simulink model "W04_P2_pid_byhand"  (R2024b)
settings: Solver=ode4  StartTime=0.0  StopTime=20  FixedStep=0.001  RelTol=1e-3
values from neighbouring files (symbols this model uses):
  Kb = 2    [W04_setup.m]
  Kd2 = evalin('base','Kd2')    [W04_pid_compare.m]    (also in W04_setup.m = 4)
  Ki2 = 8    [W04_setup.m]
  Kp2 = evalin('base','Kp2')    [W04_pid_compare.m]    (also in W04_setup.m = 10)
  Nf2 = evalin('base','Nf2')    [W04_pid_compare.m]    (also in W04_setup.m = 20)
  noise_ts = 0.01    [W04_setup.m]
  noise_var = 1e-5    (= 1e-05)    [W04_setup.m]
  plant_den = [1 2 2]    [W04_setup.m]
  plant_num = 1    [W04_setup.m]
  r_step = 1    [W04_setup.m]
  ref_smooth = 0    [W04_setup.m]
  T_ref = 0.5    [W04_setup.m]
  u_max = 2.5    [W04_setup.m]
libraries: slpidlib x1
settings Model: Creator=admin  LastModifiedBy=admin

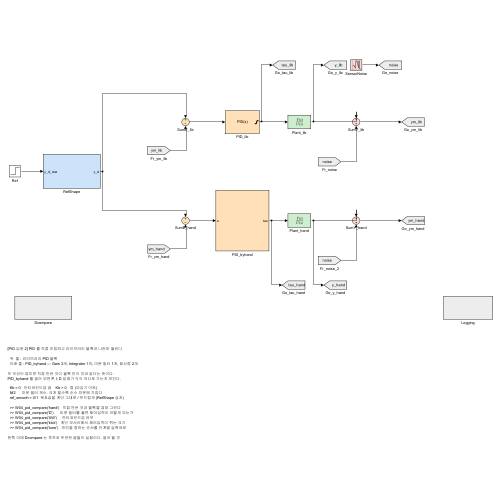
[thumbnail: Simulink's stored preview of the top-level diagram]
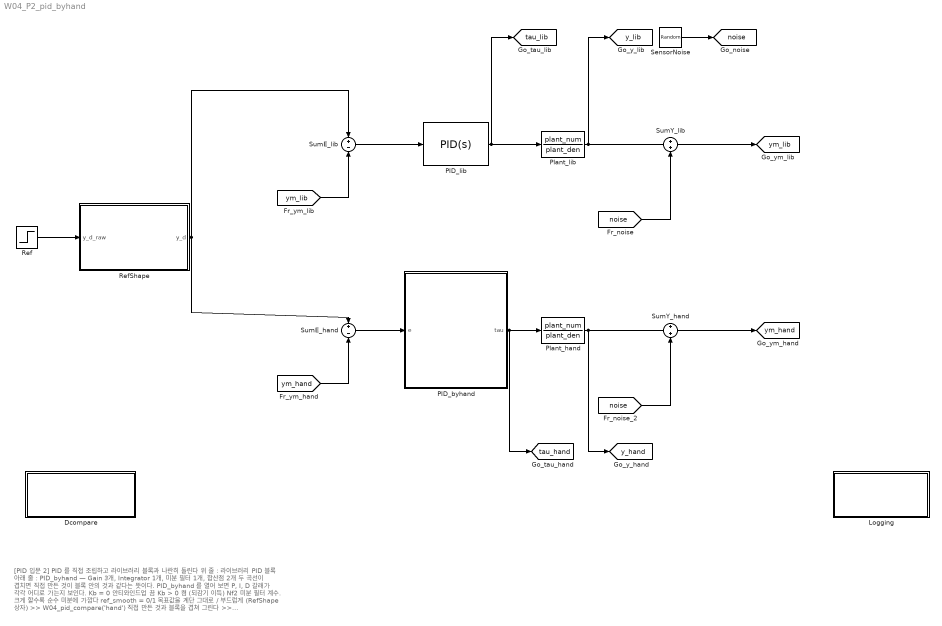
== system W04_P2_pid_byhand ==
  note: [PID 입문 2] PID 를 직접 조립하고 라이브러리 블록과 나란히 돌린다
      |
      |   위  줄 : 라이브러리 PID 블록
      |   아래 줄 : PID_byhand — Gain 3개, Integrator 1개, 미분 필터 1개, 합산점 2개
      |
      | 두 곡선이 겹치면 직접 만든 것이 블록 안의 것과 같다는 뜻이다.
      | PID_byhand 를 열어 보면 P, I, D 갈래가 각각 어디로 가는지 보인다.
      |
      |   Kb = 0   안티와인드업 끔    Kb > 0   켬 (되감기 이득)
      |   Nf2      미분 필터 계수. 크게 할수록 순수 미분에 가깝다
      |   ref_smooth = 0/1  목표값을 계단 그대로 / 부드럽게 (RefShape 상자)
      |
      |   >> W04_pid_compare('hand')   직접 만든 것과 블록을 겹쳐 그린다
      |   >> W04_pid_compare('D')      미분 필터를 풀면 제어입력이 어떻게 되는가
      |   >> W04_pid_compare('AW')     안티와인드업 유무
      |   >> W04_pid_compare('kick')   계단 모서리에서 제어입력이 튀는 크기
      |   >> W04_pid_compare('tune')   게인을 정하는 순서를 단계별 실측표로
      |
      | 왼쪽 아래 Dcompare 는 루프와 무관한 곁들이 실험이다. 열어 볼 것
  Dcompare : Subsystem
  Logging : Subsystem
  PID_byhand : Subsystem
  PID_lib : slpidlib/PID Controller  Controller=PID  Form=Parallel  TimeDomain=Continuous-time  UseExternalTs=off  SampleTime=-1  IntegratorMethod=Forward Euler  FilterMethod=Forward Euler  ControllerParametersSource=internal  P=Kp2  I=Ki2  UseKiTs=off  D=Kd2  UseExternalDerivativeSource=off  N=Nf2  UseFilter=on  TunerSelectOption=Transfer Function Based (PID Tuner App)  InitialConditionSource=internal  InitialConditionForIntegrator=0  InitialConditionForFilter=0  DifferentiatorICPrevScaledInput=0  ExternalReset=none  TrackingMode=off  Kt=1  LimitOutput=on  SatLimitsSource=internal  UpperSaturationLimit=u_max  LowerSaturationLimit=-u_max  LinearizeAsGain=on  AntiWindupMode=back-calculation  Kb=Kb  LimitIntegrator=off  UpperIntegratorSaturationLimit=inf  LowerIntegratorSaturationLimit=-inf  POutMin=[]  POutMax=[]  IOutMin=[]  IOutMax=[]  DOutMin=[]  DOutMax=[]  NOutMin=[]  NOutMax=[]  SumOutMin=[]  SumOutMax=[]  SaturationOutMin=[]  SaturationOutMax=[]  PParamMin=[]  PParamMax=[]  IParamMin=[]  IParamMax=[]  DParamMin=[]  DParamMax=[]  NParamMin=[]  NParamMax=[]  KbParamMin=[]  KbParamMax=[]  KtParamMin=[]  KtParamMax=[]  KbOutMin=[]  KbOutMax=[]  KtOutMin=[]  KtOutMax=[]  IntegratorOutMin=[]  IntegratorOutMax=[]  FilterOutMin=[]  FilterOutMax=[]  SumI1OutMin=[]  SumI1OutMax=[]  SumI2OutMin=[]  SumI2OutMax=[]  SumI3OutMin=[]  SumI3OutMax=[]  SumI4OutMin=[]  SumI4OutMax=[]  SumDOutMin=[]  SumDOutMax=[]  DifferentiatorOutMin=[]  DifferentiatorOutMax=[]  FilterDiffOutCoefMin=[]  FilterDiffOutCoefMax=[]  ReciprocalOutMin=[]  ReciprocalOutMax=[]  SumDenOutMin=[]  SumDenOutMax=[]  SumNumOutMin=[]  SumNumOutMax=[]  DivideOutMin=[]  DivideOutMax=[]  UdiffTsProdOutMin=[]  UdiffTsProdOutMax=[]  NTsProdOutMin=[]  NTsProdOutMax=[]  UintegralTsProdOutMin=[]  UintegralTsProdOutMax=[]  UngainTsProdOutMin=[]  UngainTsProdOutMax=[]  ClampingZeroOutDataTypeStr=Inherit: Inherit via back propagation  ClampingZeroOutMin=[]  ClampingZeroOutMax=[]  FilterDenConstantOutDataTypeStr=Inherit: Inherit via back propagation  FilterDenConstantOutMin=[]  FilterDenConstantOutMax=[]  PCopyOutDataTypeStr=Inherit: Inherit via back propagation  PCopyOutMin=[]  PCopyOutMax=[]  NCopyOutDataTypeStr=Inherit: Inherit via back propagation  NCopyOutMin=[]  NCopyOutMax=[]  IntegratorContinuousStateAttributes=''  IntegratorStateMustResolveToSignalObject=off  IntegratorRTWStateStorageClass=Auto  FilterContinuousStateAttributes=''  FilterStateMustResolveToSignalObject=off  FilterRTWStateStorageClass=Auto  ParallelPVariant=InternalParameters  IdealPVariant=Disabled  IVariant=InternalParameters  DVariant=InternalParameters  IntegratorVariant=Continuous  SatVariant=Enabled  AWVariant=BackCalculation  PCopyVariant=Disabled  TRVariant=Disabled  FdbkBlocksVariant=Forward  IdealPFdbkVariant=Disabled  SatFdbkVariant=Disabled  DerivativeFilterVariant=ContFilter  NVariant=InternalParameters  NCopyVariant=Disabled  FilterICVariant=InternalICsFilter  IntegratorICVariant=InternalICs  ExternalResetVariant=Disabled  TRSumVariant=Passthrough  SumFdbkVariant=Disabled  SumVariant=Sum_PID  TsampFilterVariant=InternalTs  TsampNgainVariant=Passthrough  TsampIntegralVariant=Disabled_SignalSpec  ExternalSaturationOutDataTypeStr=Inherit: Same as second input  DerivativeSourceVariant=ErrorSignal  PreIntVariant=InternalPreInt
  Plant_hand : TransferFcn  Numerator=plant_num  Denominator=plant_den
  Plant_lib : TransferFcn  Numerator=plant_num  Denominator=plant_den
  Ref : Step  After=r_step  SampleTime=0
  RefShape : Subsystem
  SensorNoise : RandomNumber  Variance=noise_var  Seed=12345  SampleTime=noise_ts
  SumE_hand : Sum  Inputs=+-
  SumE_lib : Sum  Inputs=+-
  SumY_hand : Sum
  SumY_lib : Sum
  tag scope: noise=global, tau_hand=global, tau_lib=global, y_hand=global, y_lib=global, ym_hand=global, ym_lib=global
  wires:
  SensorNoise/1 -> [noise]
  Ref/1 -> RefShape/1(y_d_raw)
  RefShape/1(y_d) -> SumE_lib/1, SumE_hand/1
  SumE_lib/1 -> PID_lib/1
  PID_lib/1 -> Plant_lib/1, [tau_lib]
  Plant_lib/1 -> SumY_lib/1, [y_lib]
  SumY_lib/1 -> [ym_lib]
  [ym_lib] -> SumE_lib/2
  [noise] -> SumY_lib/2
  SumE_hand/1 -> PID_byhand/1(e)
  PID_byhand/1(tau) -> Plant_hand/1, [tau_hand]
  Plant_hand/1 -> SumY_hand/1, [y_hand]
  SumY_hand/1 -> [ym_hand]
  [ym_hand] -> SumE_hand/2
  [noise] -> SumY_hand/2

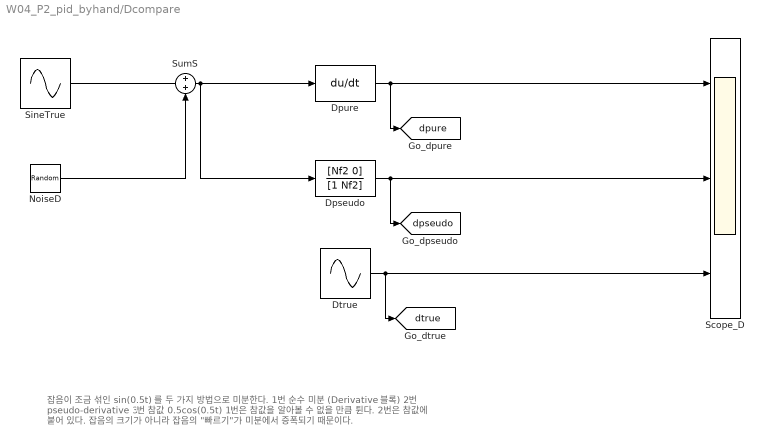
== system W04_P2_pid_byhand/Dcompare ==
  note: 잡음이 조금 섞인 sin(0.5t) 를 두 가지 방법으로 미분한다.
      |   1번 순수 미분 (Derivative 블록)     2번 pseudo-derivative     3번 참값 0.5cos(0.5t)
      | 1번은 참값을 알아볼 수 없을 만큼 튄다. 2번은 참값에 붙어 있다.
      | 잡음의 크기가 아니라 잡음의 "빠르기"가 미분에서 증폭되기 때문이다.
  Dpseudo : TransferFcn  Numerator=[Nf2 0]  Denominator=[1 Nf2]
  Dpure : Derivative
  Dtrue : Sin  Amplitude=0.5  Frequency=0.5  Phase=pi/2  SampleTime=0
  NoiseD : RandomNumber  Variance=4e-4  Seed=777  SampleTime=0.01
  Scope_D : Scope  NumInputPorts=3
  SineTrue : Sin  Frequency=0.5  SampleTime=0
  SumS : Sum
  tag scope: dpseudo=global, dpure=global, dtrue=global
  wires:
  SineTrue/1 -> SumS/1
  NoiseD/1 -> SumS/2
  SumS/1 -> Dpure/1, Dpseudo/1
  Dpure/1 -> Scope_D/1, [dpure]
  Dpseudo/1 -> Scope_D/2, [dpseudo]
  Dtrue/1 -> Scope_D/3, [dtrue]

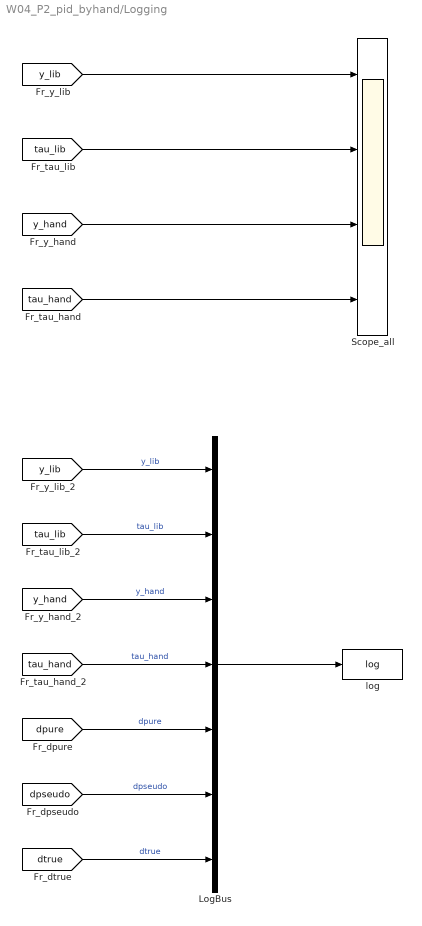
== system W04_P2_pid_byhand/Logging ==
  LogBus : BusCreator  Inputs=7
  Scope_all : Scope  NumInputPorts=4
  log : ToWorkspace  VariableName=log  SaveFormat=Timeseries  SampleTime=-1
  wires:
  [y_lib] -> Scope_all/1
  [tau_lib] -> Scope_all/2
  [y_hand] -> Scope_all/3
  [tau_hand] -> Scope_all/4
  [y_lib] -> LogBus/1  "y_lib"
  [tau_lib] -> LogBus/2  "tau_lib"
  [y_hand] -> LogBus/3  "y_hand"
  [tau_hand] -> LogBus/4  "tau_hand"
  [dpure] -> LogBus/5  "dpure"
  [dpseudo] -> LogBus/6  "dpseudo"
  [dtrue] -> LogBus/7  "dtrue"
  LogBus/1 -> log/1

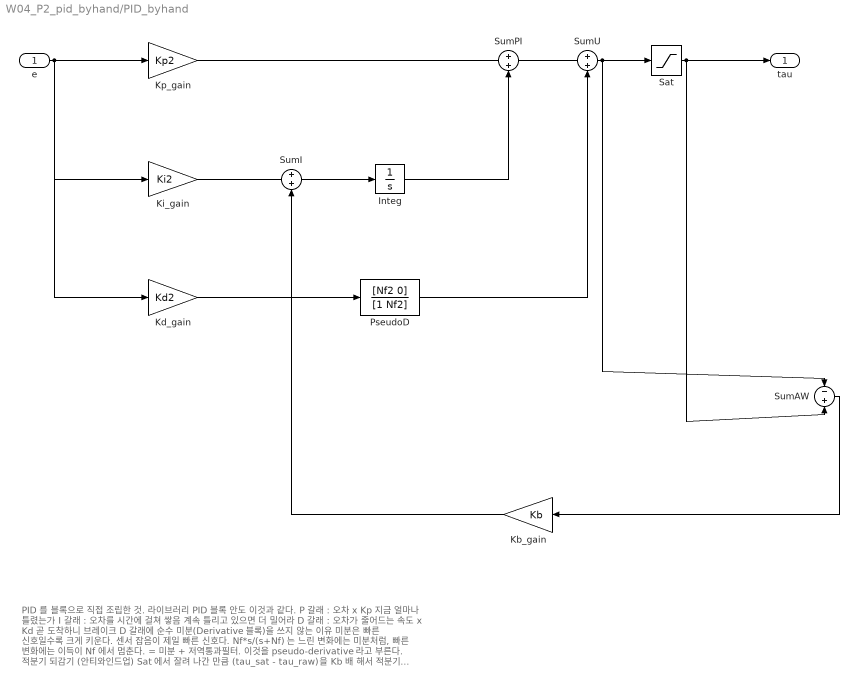
== system W04_P2_pid_byhand/PID_byhand ==
  note: PID 를 블록으로 직접 조립한 것. 라이브러리 PID 블록 안도 이것과 같다.
      |
      |   P 갈래  : 오차 x Kp                        지금 얼마나 틀렸는가
      |   I 갈래  : 오차를 시간에 걸쳐 쌓음            계속 틀리고 있으면 더 밀어라
      |   D 갈래  : 오차가 줄어드는 속도 x Kd          곧 도착하니 브레이크
      |
      | D 갈래에 순수 미분(Derivative 블록)을 쓰지 않는 이유
      |   미분은 빠른 신호일수록 크게 키운다. 센서 잡음이 제일 빠른 신호다.
      |   Nf*s/(s+Nf) 는 느린 변화에는 미분처럼, 빠른 변화에는 이득이 Nf 에서 멈춘다.
      |   = 미분 + 저역통과필터. 이것을 pseudo-derivative 라고 부른다.
      |
      | 적분기 되감기 (안티와인드업)
      |   Sat 에서 잘려 나간 만큼 (tau_sat - tau_raw) 을 Kb 배 해서 적분기 입력에 더한다.
      |   포화 중에는 이 값이 음수라 적분기가 더 쌓이지 못한다.
      |   Kb = 0 으로 두면 되감기가 사라진다. 그것이 와인드업이다.
  e : Inport
  Integ : Integrator
  Kb_gain : Gain  Gain=Kb
  Kd_gain : Gain  Gain=Kd2
  Ki_gain : Gain  Gain=Ki2
  Kp_gain : Gain  Gain=Kp2
  PseudoD : TransferFcn  Numerator=[Nf2 0]  Denominator=[1 Nf2]
  Sat : Saturate  UpperLimit=u_max  LowerLimit=-u_max
  SumAW : Sum  Inputs=-+
  SumI : Sum
  SumPI : Sum
  SumU : Sum
  tau : Outport
  wires:
  e/1 -> Kp_gain/1, Ki_gain/1, Kd_gain/1
  Ki_gain/1 -> SumI/1
  SumI/1 -> Integ/1
  Kd_gain/1 -> PseudoD/1
  Kp_gain/1 -> SumPI/1
  SumPI/1 -> SumU/1
  SumU/1 -> Sat/1, SumAW/1
  Sat/1 -> tau/1, SumAW/2
  Integ/1 -> SumPI/2
  PseudoD/1 -> SumU/2
  SumAW/1 -> Kb_gain/1
  Kb_gain/1 -> SumI/2

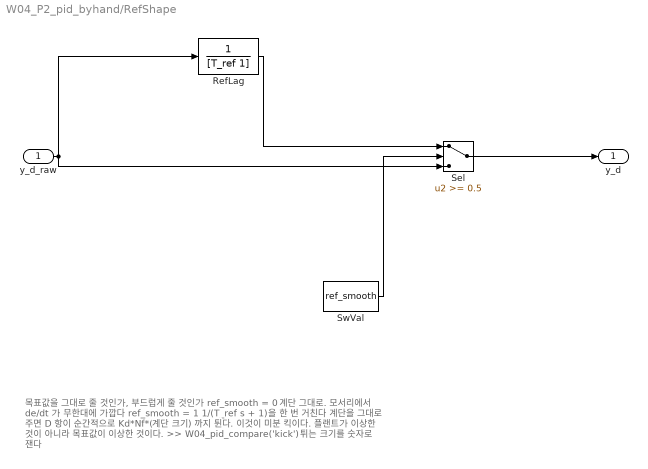
== system W04_P2_pid_byhand/RefShape ==
  note: 목표값을 그대로 줄 것인가, 부드럽게 줄 것인가
      |
      |   ref_smooth = 0   계단 그대로. 모서리에서 de/dt 가 무한대에 가깝다
      |   ref_smooth = 1   1/(T_ref s + 1) 을 한 번 거친다
      |
      | 계단을 그대로 주면 D 항이 순간적으로 Kd*Nf*(계단 크기) 까지 튄다.
      | 이것이 미분 킥이다. 플랜트가 이상한 것이 아니라 목표값이 이상한 것이다.
      |
      |   >> W04_pid_compare('kick')   튀는 크기를 숫자로 잰다
  y_d_raw : Inport
  RefLag : TransferFcn  Numerator=1  Denominator=[T_ref 1]
  Sel : Switch  Threshold=0.5  SaturateOnIntegerOverflow=off  InputSameDT=off
  SwVal : Constant  Value=ref_smooth
  y_d : Outport
  wires:
  y_d_raw/1 -> RefLag/1, Sel/3
  RefLag/1 -> Sel/1
  SwVal/1 -> Sel/2
  Sel/1 -> y_d/1
